simulink model "Prep_Matlab2_P6_MatlabBlocks"  (R2024b)
settings: Solver=VariableStepAuto  StartTime=0.0  StopTime=10  RelTol=1e-3
settings Model: Creator=yviki  LastModifiedBy=keyur
settings DebuggingCC: UnconnectedInputMsg=warning  UnconnectedOutputMsg=warning  UnconnectedLineMsg=warning
settings ModelReferenceCC: EnableRefExpFcnMdlSchedulingChecks=on
settings RTWCC: GPUComputeCapability=3.5  DLArmComputeVersion=19.05

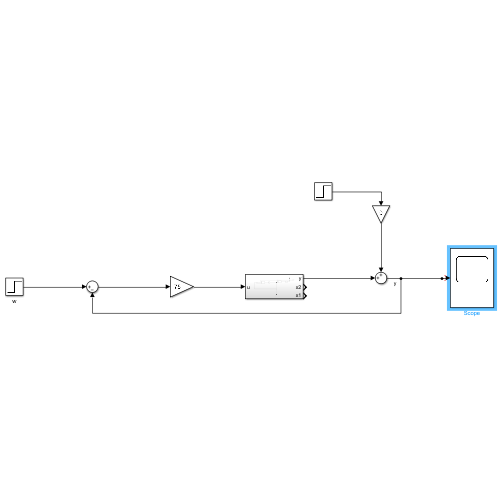
[thumbnail: Simulink's stored preview of the top-level diagram]
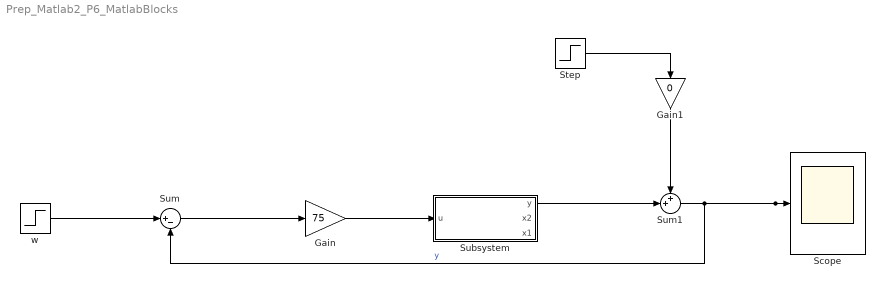
== system Prep_Matlab2_P6_MatlabBlocks ==
  Gain : Gain  Gain=75
  Gain1 : Gain  Gain=0
  Scope : Scope
  Step : Step  SampleTime=0
  Subsystem : Subsystem
  Sum : Sum  Inputs=|+-
  Sum1 : Sum  Inputs=++|
  w : Step  SampleTime=0
  wires:
  Gain/1 -> Subsystem/1(u)
  Sum/1 -> Gain/1
  Subsystem/1(y) -> Sum1/2
  Sum1/1 -> Scope/1, Sum/2  "y"
  Gain1/1 -> Sum1/1
  Step/1 -> Gain1/1
  w/1 -> Sum/1

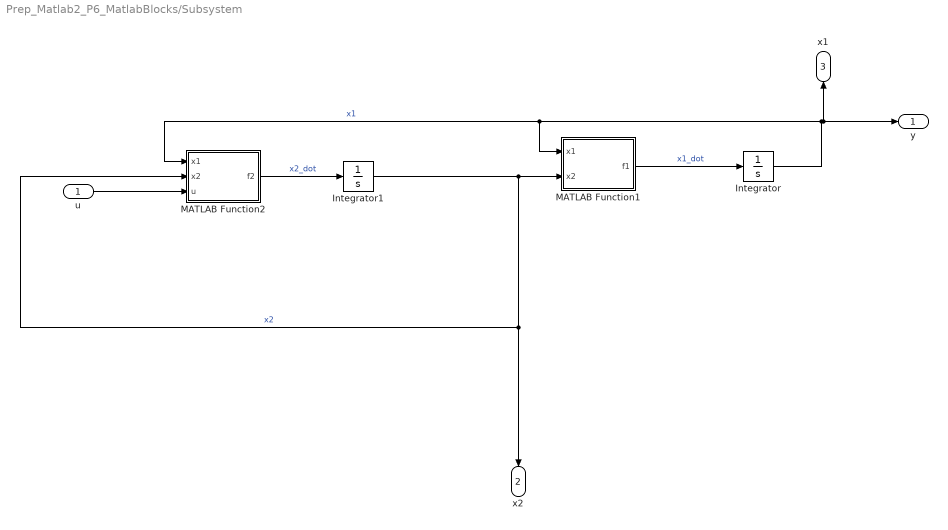
== system Prep_Matlab2_P6_MatlabBlocks/Subsystem ==
  u : Inport
  Integrator : Integrator  InitialCondition=1
  Integrator1 : Integrator  InitialCondition=1
  MATLAB Function1 : MATLAB Function  TreatAsAtomicUnit=on
  MATLAB Function2 : MATLAB Function  TreatAsAtomicUnit=on
  y : Outport
  x2 : Outport  Port=2
  x1 : Outport  Port=3
  wires:
  Integrator1/1 -> MATLAB Function2/2(x2), x2/1, MATLAB Function1/2(x2)  "x2"
  Integrator/1 -> x1/1, y/1, MATLAB Function2/1(x1), MATLAB Function1/1(x1)  "x1"
  u/1 -> MATLAB Function2/3(u)
  MATLAB Function2/1(f2) -> Integrator1/1  "x2_dot"
  MATLAB Function1/1(f1) -> Integrator/1  "x1_dot"

== matlab function Prep_Matlab2_P6_MatlabBlocks/Subsystem/MATLAB Function2 ==
  data: x1 input; f2 output; x2 input; u input
function f2 = fcn(x1, x2, u)

f2 = x1*x2 - 1 + u;

== matlab function Prep_Matlab2_P6_MatlabBlocks/Subsystem/MATLAB Function1 ==
  data: x1 input; f1 output; x2 input
function f1 = fcn(x1,x2)

f1 = -x1^3+x2;
